simulink library "mdot_DHWcalc"  (R2016b)
settings: Solver=ode45  StartTime=0.0  StopTime=10.0  RelTol=1e-3  EnableMultiTasking=on
settings Model: Creator=lena.frank  LastModifiedBy=drhf
settings DataIOCC: LimitDataPoints=on  SaveFormat=Array  SignalLoggingSaveFormat=ModelDataLogs
settings OptimizationCC: ExpressionDepthLimit=2147483647  LifeSpan=inf
settings DebuggingCC: UnderspecifiedInitializationDetection=Classic  MergeDetectMultiDrivingBlocksExec=none  SolverPrmCheckMsg=warning  FcnCallInpInsideContextMsg=warning  StateNameClashWarn=warning  SFUnexpectedBacktrackingDiag=warning  SFNoUnconditionalDefaultTransitionDiag=warning  SFExecutionAtInitializationDiag=none
settings HardwareCC: ProdBitPerPointer=32  ProdBitPerSizeT=32  ProdBitPerPtrDiffT=32  ProdLargestAtomicFloat=None  ProdIntDivRoundTo=Undefined  ProdEndianess=Unspecified  ProdWordSize=32  ProdHWDeviceType=32-bit Generic
settings ModelReferenceCC: PropagateSignalLabelsOutOfModel=off
settings GRTTargetCC: TargetLangStandard=C89/C90 (ANSI)  GeneratePreprocessorConditionals=Disable all  CombineOutputUpdateFcns=off  GRTInterface=on
settings ConfigComp: CovMetricSettings=dw  CovHtmlReporting=on  CovSaveCumulativeToWorkspaceVar=on  CovSaveSingleToWorkspaceVar=on  CovExternalEMLEnable=off

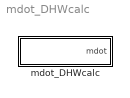
== system mdot_DHWcalc ==
  mdot_DHWcalc : Subsystem  mask(dhw from file){file=SFH_4P_200L_DHW, ext=.mat, dt=60}
      mask prompts: file "Name of file"; ext "Extension of file"; dt "Time step duration [s]"
      mask help:
      | Input for files created with the dhw-calc software.
      | These files contain only the massflow in kg/h, the conversion to kg/s is done in the block.
      | Details and manual at
      | http://solar.umwelt-uni-kassel.de/downloads.de.html
      mask init:
      | eval(['load(''' file ext ''');']);
      | eval([file ' = [ [0:dt:(length(' file ')-1)*dt]'' ' file '];' ]);
      | set_param([gcb '/dhw_from_Workspace'], 'VariableName', file);
      mask Help: eval('man (''dhw_from_file'')')
      mask TypeOptions ext: .dat | .txt | .mat | .csv
      mask Display: disp(file)

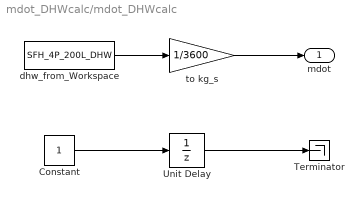
== system mdot_DHWcalc/mdot_DHWcalc ==
  Constant : Constant
  Terminator : Terminator
  Unit Delay : UnitDelay  SampleTime=dt
  dhw_from_Workspace : FromWorkspace  VariableName=SFH_4P_200L_DHW  SampleTime=0  OutputAfterFinalValue=Setting to zero
  to kg_s : Gain  Gain=1/3600
  mdot : Outport
  wires:
  to kg_s/1 -> mdot/1
  dhw_from_Workspace/1 -> to kg_s/1
  Unit Delay/1 -> Terminator/1
  Constant/1 -> Unit Delay/1
